simulink model "siasun_config_casadi_VS_lsj_sim_16a"  (R2019b)
settings: Solver=FixedStepAuto  StartTime=0.0  StopTime=20  FixedStep=0.001  RelTol=1e-3  EnableMultiTasking=on
undefined symbols (not defined in the file): a1, a2, a3, d1, d4, fc1, fc2, fc3, fc4, fc5, fc6, fv1, fv2, fv3, fv4, fv5, fv6, Ia1, Ia2, Ia3, Ia4, Ia5, Ia6, Ic111, Ic112, Ic113, Ic122, Ic123, Ic133, Ic211, Ic212, Ic213, Ic222, Ic223, Ic233, Ic311, Ic312, Ic313, Ic322, Ic323, Ic333, Ic411, Ic412, Ic413, Ic422, Ic423, Ic433, Ic511, Ic512, Ic513, Ic522, Ic523, Ic533, Ic611, Ic612, Ic613, Ic622, Ic623, Ic633, m1 ... (+26)
libraries: sm_lib x224, nesl_utility x124, simulink x8
(part 6 of 10)

== matlab function siasun_config_casadi_VS_lsj_sim_16a/Cartesian_trajectory1 ==
  data: time input; q output; initq output
function [q,initq]  = Cartesian(time)
    
    % 每次运行之前改变一下间距，再重新运行
    S = load('path.mat');
    %%  traj - 6xn
    traj = S.path;
